simulink model "scars_model_sensors"  (R2019b)
settings: Solver=FixedStepAuto  StartTime=0.0  StopTime=3500  FixedStep=dT  MaxStep=1  MinStep=dT  RelTol=1e-3
model workspace (MAT data in the model file):
  actuators = 0
values from neighbouring files (symbols this model uses):
  dtStep = 10    [SCARSSetup.m]    (also in pwsat2_setup.m; scars_setup.m)
  forcesBody = [0 0 0]    [SCARSSetup.m]    (also in pwsat2_setup.m; scars_setup.m)
  initEuler = [0 0 0]    [SCARSSetup.m]    (also in pwsat2_setup.m; scars_setup.m)
  initMoments = [0 0 0]    [SCARSSetup.m]    (also in pwsat2_setup.m; scars_setup.m)
  momentsBody = [0 0 0]    [SCARSSetup.m]    (also in pwsat2_setup.m; scars_setup.m)
  refEuler = [0 0 1]    [SCARSSetup.m]    (also in pwsat2_setup.m = [0 deg2rad(45) deg2rad(45)]; scars_setup.m)
  refVel = [v_b(1) v_b(2) v_b(3)]    [SCARSSetup.m]    (also in pwsat2_setup.m; scars_setup.m)
  stepTime = 50    [SCARSSetup.m]    (also in pwsat2_setup.m; scars_setup.m)
undefined symbols (not defined in the file or in its folder): bb, Earth, rw, WGS84
libraries: scars_library x7, aerolibgravity2 x2, aerolib6dof2 x1, sharedtransform x1, aerolibutil x1
settings Model: OrderedModelArguments=off  Creator=asmialek  LastModifiedBy=asmialek
settings DataIOCC: SaveFormat=Array  ReturnWorkspaceOutputsName=scars_out

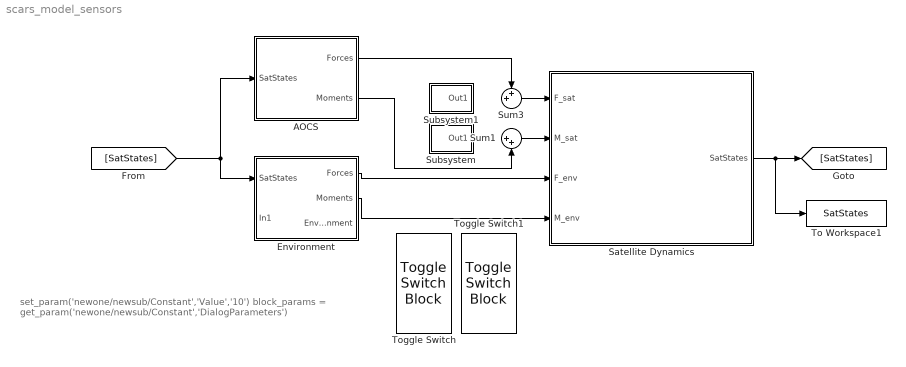
== system scars_model_sensors ==
  note: set_param('newone/newsub/Constant','Value','10')
      |
      |  block_params = get_param('newone/newsub/Constant','DialogParameters')
  AOCS : Subsystem
  Environment : Subsystem
  Satellite Dynamics : Subsystem
  Subsystem : Subsystem
  Subsystem1 : Subsystem
  Sum1 : Sum  Inputs=|++
  Sum3 : Sum  Inputs=++|
  To Workspace1 : ToWorkspace  VariableName=SatStates  SaveFormat=Timeseries  SampleTime=-1
  Toggle Switch : ToggleSwitchBlock
      settings: Values={{'Off', 'On'}, [0 1]}
  Toggle Switch1 : ToggleSwitchBlock
      settings: Values={{'Off', 'On'}, [0 1]}
  wires:
  Satellite Dynamics/1(SatStates) -> To Workspace1/1, [SatStates]
  [SatStates] -> Environment/1(SatStates), AOCS/1(SatStates)
  Environment/1(Forces) -> Satellite Dynamics/3(F_env)
  Environment/2(Moments) -> Satellite Dynamics/4(M_env)
  Sum3/1 -> Satellite Dynamics/1(F_sat)
  Sum1/1 -> Satellite Dynamics/2(M_sat)
  AOCS/1(Forces) -> Sum3/1
  AOCS/2(Moments) -> Sum1/2

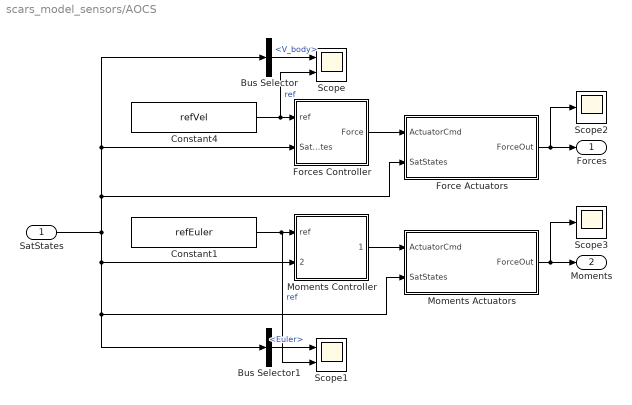
== system scars_model_sensors/AOCS ==
  SatStates : Inport
  Bus Selector : BusSelector  OutputSignals=V_body
  Bus Selector1 : BusSelector  OutputSignals=Euler
  Constant1 : Constant  Value=refEuler
  Constant4 : Constant  Value=refVel
  Force Actuators : Subsystem  mask{ActuatorType=Thrusters}
      mask prompts: ActuatorType "Actuator Type"
      mask TypeOptions ActuatorType: Thrusters | None
      mask Callback ActuatorType:
      | value = get_param(gcb,'ActuatorType');
      | % disp(value);
      | if strcmp(value,'Perfect')
      |     assignin('base','actuators',1)
      | elseif strcmp(value,'Thrusters')
      |     assignin('base','actuators',2)
      | elseif strcmp(value,'None')
      |     assignin('base','actuators',4)
      | else
      |     assignin('base','actuators',4)
      | end
  Forces Controller : Subsystem
  Moments Actuators : Subsystem  mask{ActuatorType=Thrusters}
      mask prompts: ActuatorType "Actuator Type"
      mask TypeOptions ActuatorType: Thrusters | None
      mask Callback ActuatorType:
      | value = get_param(gcb,'ActuatorType');
      | % disp(value);
      | if strcmp(value,'Perfect')
      |     assignin('base','actuators',1)
      | elseif strcmp(value,'Thrusters')
      |     assignin('base','actuators',2)
      | elseif strcmp(value,'None')
      |     assignin('base','actuators',4)
      | else
      |     assignin('base','actuators',4)
      | end
  Moments Controller : Subsystem
  Scope : Scope  NumInputPorts=2
  Scope1 : Scope  NumInputPorts=2
  Scope2 : Scope
  Scope3 : Scope
  Forces : Outport
  Moments : Outport  Port=2
  wires:
  Moments Controller/1(Torque) -> Moments Actuators/1(ActuatorCmd)
  Force Actuators/1(ForceOut) -> Scope2/1, Forces/1
  SatStates/1 -> Bus Selector1/1, Moments Actuators/2(SatStates), Moments Controller/2(SatStates), Bus Selector/1, Forces Controller/2(SatStates), Force Actuators/2(SatStates)
  Constant4/1 -> Scope/2, Forces Controller/1(ref)  "ref"
  Forces Controller/1(Force) -> Force Actuators/1(ActuatorCmd)
  Constant1/1 -> Scope1/2, Moments Controller/1(ref)  "ref"
  Bus Selector/1 -> Scope/1  "<V_body>"
  Bus Selector1/1 -> Scope1/1  "<Euler>"
  Moments Actuators/1(ForceOut) -> Scope3/1, Moments/1

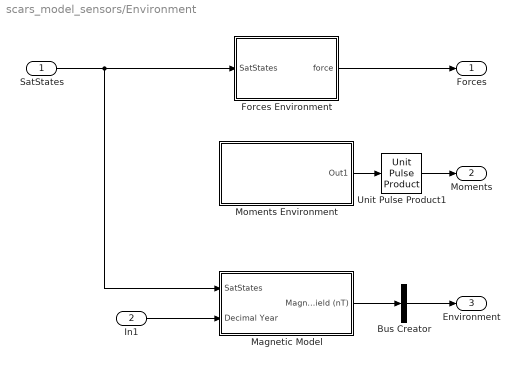
== system scars_model_sensors/Environment ==
  SatStates : Inport
  In1 : Inport  Port=2
  Bus Creator : BusCreator  Inputs=1
  Forces Environment : Subsystem
  Magnetic Model : Subsystem
  Moments Environment : Subsystem
  Unit Pulse Product1 : scars_library/Unit Pulse Product  startTime=stepTime  length=dtStep
  Forces : Outport
  Moments : Outport  Port=2
  Environment : Outport  Port=3
  wires:
  Moments Environment/1(Out1) -> Unit Pulse Product1/1
  SatStates/1 -> Magnetic Model/1(SatStates), Forces Environment/1(SatStates)
  Forces Environment/1(force) -> Forces/1
  Unit Pulse Product1/1 -> Moments/1
  Magnetic Model/1(Magnetic Field (nT)) -> Bus Creator/1
  Bus Creator/1 -> Environment/1
  In1/1 -> Magnetic Model/2(Decimal Year)

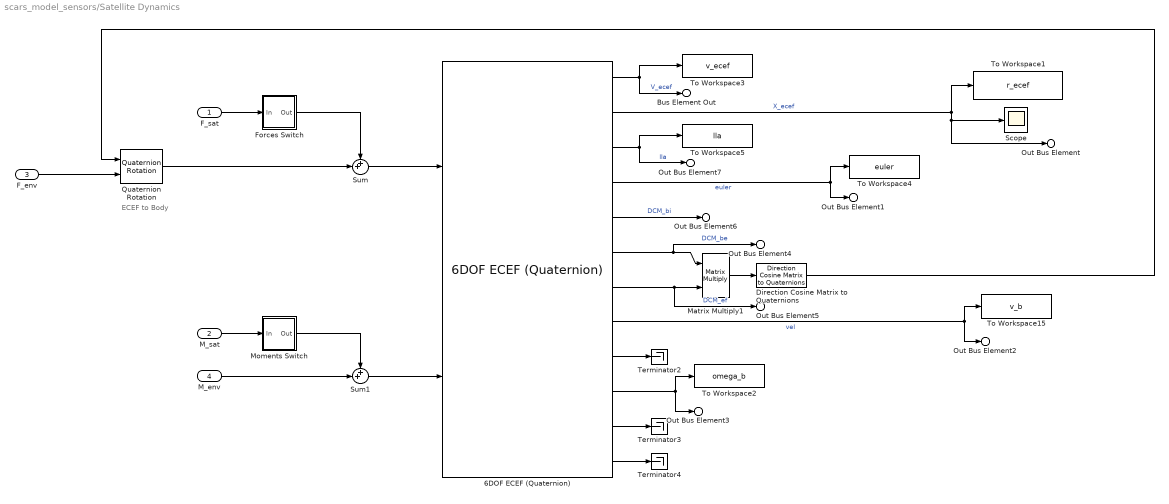
== system scars_model_sensors/Satellite Dynamics ==
  note: ECEF to Body
  F_sat : Inport
  M_sat : Inport  Port=2
  F_env : Inport  Port=3
  M_env : Inport  Port=4
  6DOF ECEF (Quaternion) : aerolib6dof2/6DOF ECEF (Quaternion)  units=Metric (MKS)  mtype=Fixed  xg_0=r_lla  Vm_0=v_b  eul_0=deg2rad(initEuler)  pm_0=[0 0 0]  mass_0=1.0  mass_e=0.5  mass_f=2.0  inertia=eye(3)  inertia_e=eye(3)  inertia_f=2*eye(3)  vre_flag=on  abi_flag=off  ptype=Earth (WGS84)  R=6378137  F=1/298.257223563  w_E=7292115e-11  angle_in=Internal  LG0=0  quat_statename=''  pm_statename=''  Vm_statename=''  posECEF_statename=''  posECI_statename=''  LG_statename=''  mass_statename=''
      settings: SourceProductName=Aerospace Blockset  SourceProductBaseCode=AE
  Direction Cosine Matrix to Quaternions : sharedtransform/Direction Cosine Matrix  to Quaternions  aMode=0  action=None  tolerance=eps(2)
      settings: SourceProductName=Aerospace Blockset  SourceProductBaseCode=AE
  Forces Switch : Subsystem
  Matrix Multiply1 : Product  Multiplication=Matrix(*)
  Moments Switch : Subsystem
  Quaternion Rotation : aerolibutil/Quaternion Rotation
  Scope : Scope
  Sum : Sum  Inputs=++|
  Sum1 : Sum  Inputs=++|
  Terminator2 : Terminator
  Terminator3 : Terminator
  Terminator4 : Terminator
  To Workspace1 : ToWorkspace  VariableName=r_ecef  SampleTime=-1
  To Workspace15 : ToWorkspace  VariableName=v_b  SampleTime=-1
      settings: Save2DSignal=2-D array (concatenate along first dimension)
  To Workspace2 : ToWorkspace  VariableName=omega_b  SampleTime=-1
      settings: Save2DSignal=2-D array (concatenate along first dimension)
  To Workspace3 : ToWorkspace  VariableName=v_ecef  SampleTime=-1
      settings: Save2DSignal=2-D array (concatenate along first dimension)
  To Workspace4 : ToWorkspace  VariableName=euler  SampleTime=-1
      settings: Save2DSignal=2-D array (concatenate along first dimension)
  To Workspace5 : ToWorkspace  VariableName=lla  SampleTime=-1
      settings: Save2DSignal=2-D array (concatenate along first dimension)
  Bus Element Out : Outport  PortName=SatStates  Element=V_ecef
  Out Bus Element : Outport  PortName=SatStates  Element=X_ecef
  Out Bus Element1 : Outport  PortName=SatStates  Element=Euler
  Out Bus Element2 : Outport  PortName=SatStates  Element=V_body
  Out Bus Element3 : Outport  PortName=SatStates  Element=Omega_body
  Out Bus Element6 : Outport  PortName=SatStates  Element=ECI2Body
  Out Bus Element4 : Outport  PortName=SatStates  Element=NED2Body
  Out Bus Element5 : Outport  PortName=SatStates  Element=ECEF2NED
  Out Bus Element7 : Outport  PortName=SatStates  Element=lla
  wires:
  6DOF ECEF (Quaternion)/1 -> To Workspace3/1, Bus Element Out/1  "V_ecef"
  6DOF ECEF (Quaternion)/8 -> Out Bus Element2/1, To Workspace15/1  "vel"
  6DOF ECEF (Quaternion)/2 -> Scope/1, Out Bus Element/1, To Workspace1/1  "X_ecef"
  6DOF ECEF (Quaternion)/6 -> Out Bus Element4/1, Matrix Multiply1/1  "DCM_be"
  Sum/1 -> 6DOF ECEF (Quaternion)/1
  6DOF ECEF (Quaternion)/7 -> Out Bus Element5/1, Matrix Multiply1/2  "DCM_ef"
  6DOF ECEF (Quaternion)/4 -> Out Bus Element1/1, To Workspace4/1  "euler"
  6DOF ECEF (Quaternion)/10 -> To Workspace2/1, Out Bus Element3/1
  M_env/1 -> Sum1/2
  Sum1/1 -> 6DOF ECEF (Quaternion)/2
  Matrix Multiply1/1 -> Direction Cosine Matrix to Quaternions/1
  F_sat/1 -> Forces Switch/1(In)
  Quaternion Rotation/1 -> Sum/2
  F_env/1 -> Quaternion Rotation/2
  Direction Cosine Matrix to Quaternions/1 -> Quaternion Rotation/1
  Forces Switch/1(Out) -> Sum/1
  M_sat/1 -> Moments Switch/1(In)
  Moments Switch/1(Out) -> Sum1/1
  6DOF ECEF (Quaternion)/5 -> Out Bus Element6/1  "DCM_bi"
  6DOF ECEF (Quaternion)/9 -> Terminator2/1
  6DOF ECEF (Quaternion)/11 -> Terminator3/1
  6DOF ECEF (Quaternion)/12 -> Terminator4/1
  6DOF ECEF (Quaternion)/3 -> Out Bus Element7/1, To Workspace5/1  "lla"

== system scars_model_sensors/Subsystem ==
  Constant1 : Constant  Value=momentsBody
  Constant2 : Constant  Value=momentsBody
  Gain : Gain  Gain=-1
  Sum : Sum  Inputs=|++
  Unit Pulse Product1 : scars_library/Unit Pulse Product  startTime=stepTime  length=dtStep
  Unit Pulse Product2 : scars_library/Unit Pulse Product  startTime=stepTime+dtStep  length=dtStep
  Out1 : Outport
  wires:
  Constant1/1 -> Unit Pulse Product1/1
  Unit Pulse Product1/1 -> Sum/1
  Sum/1 -> Out1/1
  Constant2/1 -> Unit Pulse Product2/1
  Gain/1 -> Sum/2
  Unit Pulse Product2/1 -> Gain/1

== system scars_model_sensors/Subsystem1 ==
  Constant2 : Constant  Value=forcesBody
  Unit Pulse Product : scars_library/Unit Pulse Product  startTime=stepTime+100  length=dtStep
  Out1 : Outport
  wires:
  Constant2/1 -> Unit Pulse Product/1
  Unit Pulse Product/1 -> Out1/1

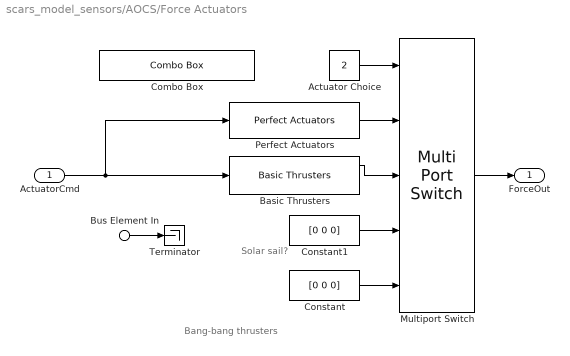
== system scars_model_sensors/AOCS/Force Actuators ==
  note: Bang-bang thrusters
  note: Solar sail?
  ActuatorCmd : Inport
  Bus Element In : Inport  Port=2  PortName=SatStates  Element=V_ecef
  Actuator Choice : Constant  Value=2
  Basic Thrusters : scars_library/Basic Thrusters  SystemSampleTime=-1  Latency=0  AutoFrameSizeCalculation=off
  Combo Box : ComboBox  LabelPosition=Hide  SelectedLabel=Thrusters
      settings: Values={{'Perfect Actuators', 'Thrusters', 'idontknowyet', 'No Actuators'}, [1 2 3 4]}
  Constant : Constant  Value=[0 0 0]
  Constant1 : Constant  Value=[0 0 0]
  Multiport Switch : MultiPortSwitch  Inputs=4  DiagnosticForDefault=Warning
  Perfect Actuators : scars_library/Perfect Actuators  Parameter1=on
  Terminator : Terminator
  ForceOut : Outport
  wires:
  Perfect Actuators/1 -> Multiport Switch/2
  Constant/1 -> Multiport Switch/5
  Actuator Choice/1 -> Multiport Switch/1
  Basic Thrusters/1 -> Multiport Switch/3
  ActuatorCmd/1 -> Basic Thrusters/1, Perfect Actuators/1
  Multiport Switch/1 -> ForceOut/1
  Constant1/1 -> Multiport Switch/4
  Bus Element In/1 -> Terminator/1

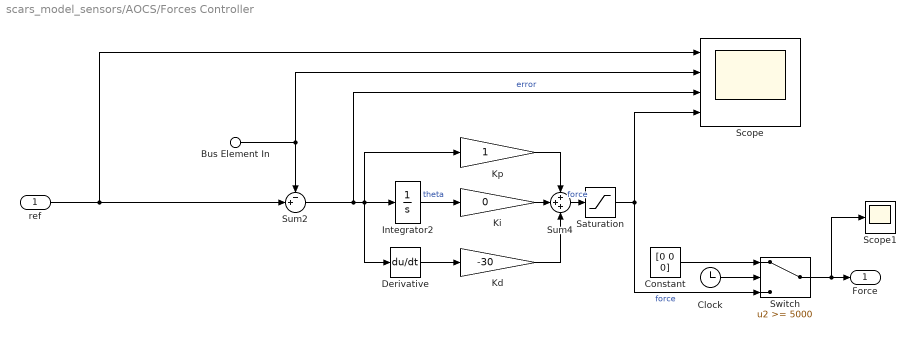
== system scars_model_sensors/AOCS/Forces Controller ==
  ref : Inport
  Bus Element In : Inport  Port=2  PortName=SatStates  Element=V_body
  Clock : Clock
  Constant : Constant  Value=[0 0 0]
  Derivative : Derivative
  Integrator2 : Integrator
  Kd : Gain  Gain=-30
  Ki : Gain  Gain=0
  Kp : Gain
  Saturation : Saturate
  Scope : Scope  NumInputPorts=4
  Scope1 : Scope
  Sum2 : Sum  Inputs=-+|
  Sum4 : Sum  Inputs=+++
  Switch : Switch  Threshold=5000
  Force : Outport
  wires:
  Saturation/1 -> Switch/3, Scope/4  "force"
  ref/1 -> Sum2/2, Scope/1
  Clock/1 -> Switch/2
  Switch/1 -> Scope1/1, Force/1
  Constant/1 -> Switch/1
  Bus Element In/1 -> Sum2/1, Scope/2
  Integrator2/1 -> Ki/1  "theta"
  Kp/1 -> Sum4/1
  Sum2/1 -> Kp/1, Derivative/1, Integrator2/1, Scope/3  "error"
  Kd/1 -> Sum4/3
  Ki/1 -> Sum4/2
  Derivative/1 -> Kd/1
  Sum4/1 -> Saturation/1  "force"

== system scars_model_sensors/AOCS/Moments Actuators ==
  ActuatorCmd : Inport
  Bus Element In : Inport  Port=2  PortName=SatStates  Element=Euler
  Actuator Choice : Constant  Value=2
  Bang-Bang Thrusters : Subsystem
  Constant : Constant  Value=[0 0 0]
  Multiport Switch : MultiPortSwitch  Inputs=4  DiagnosticForDefault=Warning
  Perfect Actuators : scars_library/Perfect Actuators  Parameter1=on
  Reaction Wheels : Subsystem
  ForceOut : Outport
  wires:
  Perfect Actuators/1 -> Multiport Switch/2
  Constant/1 -> Multiport Switch/5
  Actuator Choice/1 -> Multiport Switch/1
  Bang-Bang Thrusters/1(Torque) -> Multiport Switch/3
  Reaction Wheels/1(Torque) -> Multiport Switch/4
  Multiport Switch/1 -> ForceOut/1
  ActuatorCmd/1 -> Bang-Bang Thrusters/1(TorqueCmd), Perfect Actuators/1, Reaction Wheels/2(TorqueCmd)
  Bus Element In/1 -> Reaction Wheels/1(Euler)

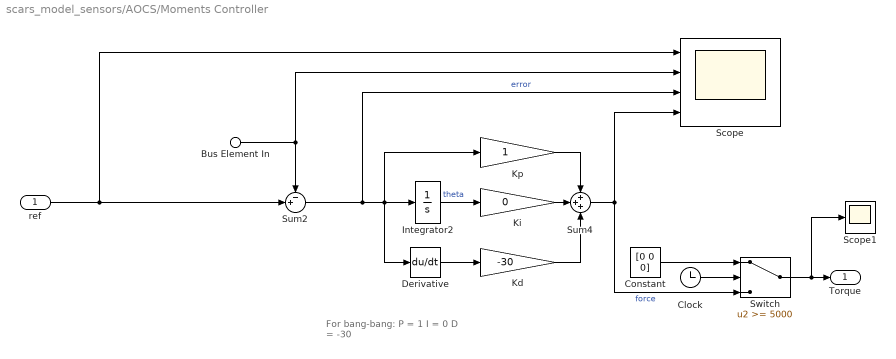
== system scars_model_sensors/AOCS/Moments Controller ==
  note: For bang-bang:
      | P = 1
      | I = 0
      | D = -30
  ref : Inport
  Bus Element In : Inport  Port=2  PortName=SatStates  Element=Euler
  Clock : Clock
  Constant : Constant  Value=[0 0 0]
  Derivative : Derivative
  Integrator2 : Integrator
  Kd : Gain  Gain=-30
  Ki : Gain  Gain=0
  Kp : Gain
  Scope : Scope  NumInputPorts=4
  Scope1 : Scope
  Sum2 : Sum  Inputs=-+|
  Sum4 : Sum  Inputs=+++
  Switch : Switch  Threshold=5000
  Torque : Outport
  wires:
  Sum4/1 -> Switch/3, Scope/4  "force"
  ref/1 -> Sum2/2, Scope/1
  Clock/1 -> Switch/2
  Switch/1 -> Scope1/1, Torque/1
  Constant/1 -> Switch/1
  Bus Element In/1 -> Sum2/1, Scope/2
  Derivative/1 -> Kd/1
  Kd/1 -> Sum4/3
  Ki/1 -> Sum4/2
  Integrator2/1 -> Ki/1  "theta"
  Sum2/1 -> Kp/1, Derivative/1, Integrator2/1, Scope/3  "error"
  Kp/1 -> Sum4/1

== system scars_model_sensors/Environment/Forces Environment ==
  Bus Element In : Inport  PortName=SatStates  Element=X_ecef
  Spherical Harmonic Gravity Model1 : aerolibgravity2/Spherical Harmonic Gravity Model  units=Metric (MKS)  degree=120  action=Warning  ptype=EGM2008  datafile='aerogmm2b.mat'
      settings: SourceProductName=Aerospace Blockset  SourceProductBaseCode=AE
  To Workspace13 : ToWorkspace  VariableName=g  SampleTime=-1
  force : Outport
  wires:
  Spherical Harmonic Gravity Model1/1 -> force/1, To Workspace13/1
  Bus Element In/1 -> Spherical Harmonic Gravity Model1/1

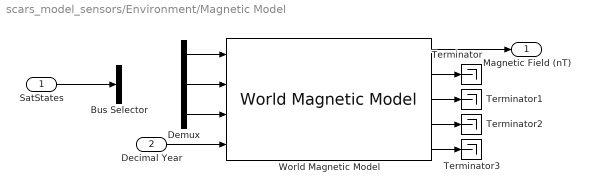
== system scars_model_sensors/Environment/Magnetic Model ==
  SatStates : Inport
  Decimal Year : Inport  Port=2
  Bus Selector : BusSelector  OutputSignals=signal1,signal2
  Demux : Demux  Outputs=3
  Terminator{,1..3} (4 alike) : Terminator
  World Magnetic Model : aerolibgravity2/World Magnetic Model  model=WMM2015 V2 (2015-2020)  customFile='WMM2015v2.COF'  units=Metric (MKS)  time_in=on  month=January  day=1  year=2015  action=Error  h_out=on  dec_out=on  inc_out=on  ti_out=on
      settings: SourceProductName=Aerospace Blockset  SourceProductBaseCode=AE
  Magnetic Field (nT) : Outport
  wires:
  World Magnetic Model/4 -> Terminator2/1
  Demux/1 -> World Magnetic Model/1
  World Magnetic Model/1 -> Magnetic Field (nT)/1
  Demux/3 -> World Magnetic Model/3
  Decimal Year/1 -> World Magnetic Model/4
  World Magnetic Model/2 -> Terminator/1
  World Magnetic Model/5 -> Terminator3/1
  World Magnetic Model/3 -> Terminator1/1
  Demux/2 -> World Magnetic Model/2
  SatStates/1 -> Bus Selector/1

== system scars_model_sensors/Environment/Moments Environment ==
  Constant : Constant  Value=initMoments
  Out1 : Outport
  wires:
  Constant/1 -> Out1/1

== system scars_model_sensors/Satellite Dynamics/Forces Switch ==
  In : Inport
  Constant1 : Constant  Value=[0 0 0]
  Forces : Constant  Value=0
  Switch : Switch  Criteria=u2 > Threshold
  Out : Outport
  wires:
  Constant1/1 -> Switch/3
  Forces/1 -> Switch/2
  Switch/1 -> Out/1
  In/1 -> Switch/1

== system scars_model_sensors/Satellite Dynamics/Moments Switch ==
  In : Inport
  Constant1 : Constant  Value=[0 0 0]
  Moments : Constant  Value=0
  Switch : Switch  Criteria=u2 > Threshold
  Out : Outport
  wires:
  In/1 -> Switch/1
  Constant1/1 -> Switch/3
  Switch/1 -> Out/1
  Moments/1 -> Switch/2

== system scars_model_sensors/AOCS/Moments Actuators/Bang-Bang Thrusters ==
  TorqueCmd : Inport
  Demux : Demux  Outputs=3
  Gain : Gain  Gain=-1
  Mux : Mux  Inputs=3
  Thruster Pitch : Subsystem
  Thruster Roll : Subsystem
  Thruster Yaw : Subsystem
  Torque : Outport  VectorParamsAs1DForOutWhenUnconnected=off
  wires:
  Thruster Roll/1(Torque Out) -> Mux/1
  Thruster Pitch/1(Torque Out) -> Mux/2
  Thruster Yaw/1(Torque Out) -> Mux/3
  TorqueCmd/1 -> Demux/1
  Demux/2 -> Thruster Pitch/1(Torque)
  Demux/1 -> Thruster Roll/1(Torque)
  Demux/3 -> Thruster Yaw/1(Torque)
  Mux/1 -> Gain/1
  Gain/1 -> Torque/1

== system scars_model_sensors/AOCS/Moments Actuators/Reaction Wheels ==
  Euler : Inport
  TorqueCmd : Inport  Port=2
  Demux : Demux  Outputs=3
  Demux2 : Demux  Outputs=3
  Mux : Mux  Inputs=3
  Reaction Wheel Pitch : Subsystem
  Reaction Wheel Roll : Subsystem
  Reaction Wheel Yaw : Subsystem
  Torque : Outport  VectorParamsAs1DForOutWhenUnconnected=off
  wires:
  Mux/1 -> Torque/1
  Demux/1 -> Reaction Wheel Roll/2(Torque)
  Reaction Wheel Roll/1(Torque Out) -> Mux/1
  Demux2/1 -> Reaction Wheel Roll/1(Rate)
  Demux2/2 -> Reaction Wheel Pitch/1(Rate)
  Demux/2 -> Reaction Wheel Pitch/2(Torque)
  Demux2/3 -> Reaction Wheel Yaw/1(Rate)
  Demux/3 -> Reaction Wheel Yaw/2(Torque)
  Reaction Wheel Pitch/1(Torque Out) -> Mux/2
  Reaction Wheel Yaw/1(Torque Out) -> Mux/3
  Euler/1 -> Demux2/1
  TorqueCmd/1 -> Demux/1

== system scars_model_sensors/AOCS/Moments Actuators/Bang-Bang Thrusters/Thruster Pitch ==
  Torque : Inport
  Gain2 : Gain  Gain=-1
  Relay1 : Relay  OnSwitchValue=bb.a1  OffSwitchValue=bb.a0  OnOutputValue=bb.thrust
  Relay2 : Relay  OnSwitchValue=bb.a1  OffSwitchValue=bb.a0  OnOutputValue=-bb.thrust
  Scope1 : Scope  NumInputPorts=5
  Sum1 : Sum  Inputs=-|-
  Sum2 : Sum  Inputs=+|+
  Torque Out : Outport
  wires:
  Sum1/1 -> Torque Out/1  "M"
  Relay2/1 -> Scope1/3, Sum2/2
  Sum2/1 -> Scope1/5, Sum1/1
  Gain2/1 -> Scope1/2, Relay2/1
  Relay1/1 -> Scope1/4, Sum2/1
  Torque/1 -> Scope1/1, Relay1/1, Gain2/1  "pd"

== system scars_model_sensors/AOCS/Moments Actuators/Bang-Bang Thrusters/Thruster Roll ==
  Torque : Inport
  Gain2 : Gain  Gain=-1
  Relay1 : Relay  OnSwitchValue=bb.a1  OffSwitchValue=bb.a0  OnOutputValue=bb.thrust
  Relay2 : Relay  OnSwitchValue=bb.a1  OffSwitchValue=bb.a0  OnOutputValue=-bb.thrust
  Scope1 : Scope  NumInputPorts=5
  Sum1 : Sum  Inputs=-|-
  Sum2 : Sum  Inputs=+|+
  Torque Out : Outport
  wires:
  Sum1/1 -> Torque Out/1  "M"
  Relay2/1 -> Scope1/3, Sum2/2
  Sum2/1 -> Scope1/5, Sum1/1
  Gain2/1 -> Scope1/2, Relay2/1
  Relay1/1 -> Scope1/4, Sum2/1
  Torque/1 -> Scope1/1, Relay1/1, Gain2/1  "pd"

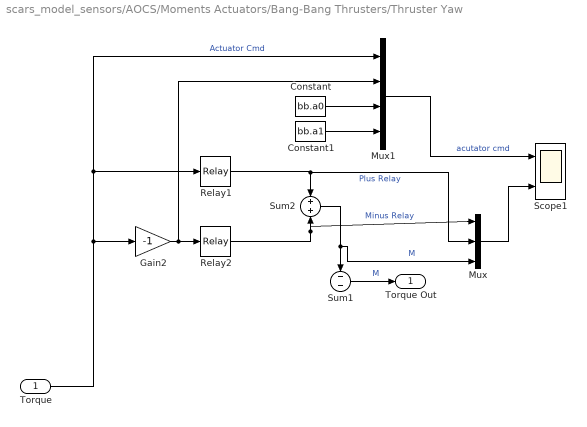
== system scars_model_sensors/AOCS/Moments Actuators/Bang-Bang Thrusters/Thruster Yaw ==
  Torque : Inport
  Constant : Constant  Value=bb.a0
  Constant1 : Constant  Value=bb.a1
  Gain2 : Gain  Gain=-1
  Mux : Mux  Inputs=3
  Mux1 : Mux
  Relay1 : Relay  OnSwitchValue=bb.a1  OffSwitchValue=bb.a0  OnOutputValue=bb.thrust
  Relay2 : Relay  OnSwitchValue=bb.a1  OffSwitchValue=bb.a0  OnOutputValue=-bb.thrust
  Scope1 : Scope  NumInputPorts=2
  Sum1 : Sum  Inputs=-|-
  Sum2 : Sum  Inputs=+|+
  Torque Out : Outport
  wires:
  Sum1/1 -> Torque Out/1  "M"
  Relay2/1 -> Mux/1, Sum2/2  "Minus Relay"
  Sum2/1 -> Mux/3, Sum1/1  "M"
  Gain2/1 -> Mux1/2, Relay2/1
  Relay1/1 -> Mux/2, Sum2/1  "Plus Relay"
  Torque/1 -> Relay1/1, Mux1/1, Gain2/1  "Actuator Cmd"
  Mux1/1 -> Scope1/1  "acutator cmd"
  Mux/1 -> Scope1/2
  Constant/1 -> Mux1/3
  Constant1/1 -> Mux1/4

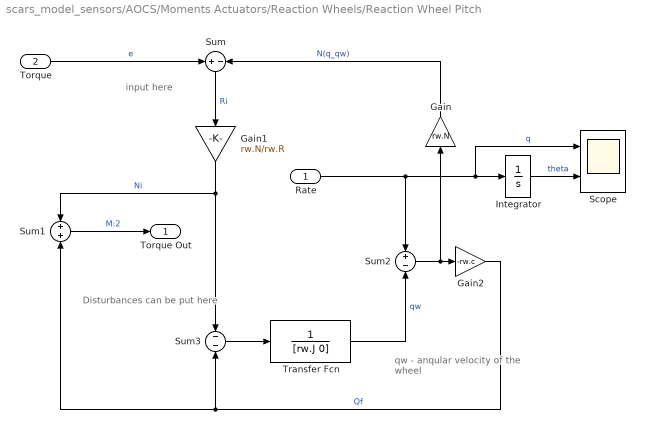
== system scars_model_sensors/AOCS/Moments Actuators/Reaction Wheels/Reaction Wheel Pitch ==
  note: qw - anqular velocity
      |  of the wheel
  note: input here
  note: Disturbances can
      | be put here
  Rate : Inport
  Torque : Inport  Port=2
  Gain : Gain  Gain=rw.N
  Gain1 : Gain  Gain=rw.N/rw.R
  Gain2 : Gain  Gain=-rw.c
  Integrator : Integrator
  Scope : Scope  NumInputPorts=2
  Sum : Sum  Inputs=+|-
  Sum1 : Sum  Inputs=+|+
  Sum2 : Sum  Inputs=+|-
  Sum3 : Sum  Inputs=-|-
  Transfer Fcn : TransferFcn  Denominator=[rw.J 0]
  Torque Out : Outport
  wires:
  Gain2/1 -> Sum1/2, Sum3/2  "Qf"
  Gain1/1 -> Sum1/1, Sum3/1  "Ni"
  Integrator/1 -> Scope/2  "theta"
  Sum3/1 -> Transfer Fcn/1
  Torque/1 -> Sum/1  "e"
  Sum1/1 -> Torque Out/1  "M:2"
  Gain/1 -> Sum/2  "N(q_qw)"
  Rate/1 -> Sum2/1, Integrator/1, Scope/1  "q"
  Sum2/1 -> Gain/1, Gain2/1
  Sum/1 -> Gain1/1  "Ri"
  Transfer Fcn/1 -> Sum2/2  "qw"

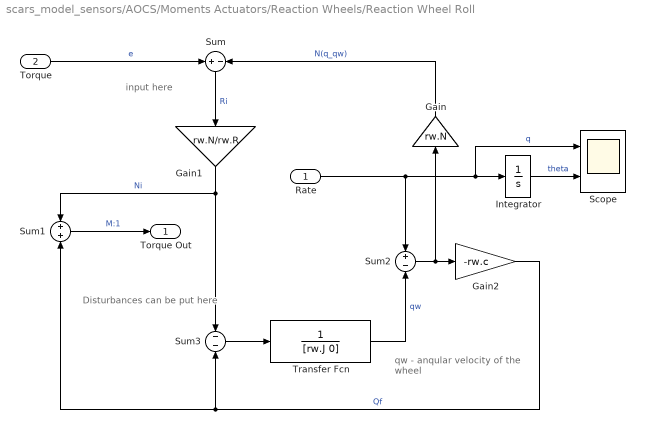
== system scars_model_sensors/AOCS/Moments Actuators/Reaction Wheels/Reaction Wheel Roll ==
  note: Disturbances can
      | be put here
  note: input here
  note: qw - anqular velocity
      |  of the wheel
  Rate : Inport
  Torque : Inport  Port=2
  Gain : Gain  Gain=rw.N
  Gain1 : Gain  Gain=rw.N/rw.R
  Gain2 : Gain  Gain=-rw.c
  Integrator : Integrator
  Scope : Scope  NumInputPorts=2
  Sum : Sum  Inputs=+|-
  Sum1 : Sum  Inputs=+|+
  Sum2 : Sum  Inputs=+|-
  Sum3 : Sum  Inputs=-|-
  Transfer Fcn : TransferFcn  Denominator=[rw.J 0]
  Torque Out : Outport
  wires:
  Gain1/1 -> Sum1/1, Sum3/1  "Ni"
  Torque/1 -> Sum/1  "e"
  Sum3/1 -> Transfer Fcn/1
  Sum/1 -> Gain1/1  "Ri"
  Integrator/1 -> Scope/2  "theta"
  Transfer Fcn/1 -> Sum2/2  "qw"
  Gain2/1 -> Sum1/2, Sum3/2  "Qf"
  Sum1/1 -> Torque Out/1  "M:1"
  Sum2/1 -> Gain2/1, Gain/1
  Gain/1 -> Sum/2  "N(q_qw)"
  Rate/1 -> Sum2/1, Integrator/1, Scope/1  "q"

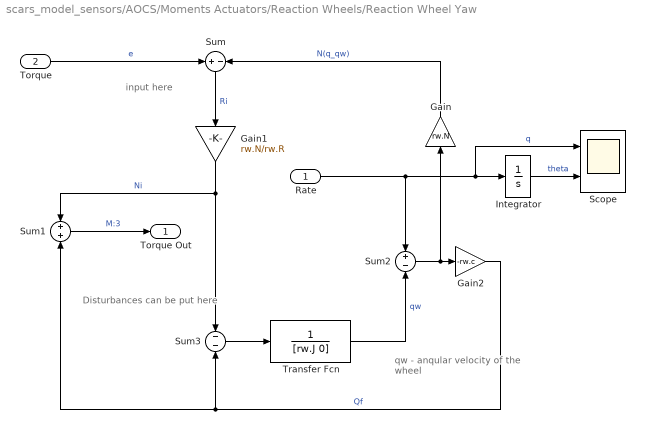
== system scars_model_sensors/AOCS/Moments Actuators/Reaction Wheels/Reaction Wheel Yaw ==
  note: qw - anqular velocity
      |  of the wheel
  note: input here
  note: Disturbances can
      | be put here
  Rate : Inport
  Torque : Inport  Port=2
  Gain : Gain  Gain=rw.N
  Gain1 : Gain  Gain=rw.N/rw.R
  Gain2 : Gain  Gain=-rw.c
  Integrator : Integrator
  Scope : Scope  NumInputPorts=2
  Sum : Sum  Inputs=+|-
  Sum1 : Sum  Inputs=+|+
  Sum2 : Sum  Inputs=+|-
  Sum3 : Sum  Inputs=-|-
  Transfer Fcn : TransferFcn  Denominator=[rw.J 0]
  Torque Out : Outport
  wires:
  Gain2/1 -> Sum1/2, Sum3/2  "Qf"
  Gain1/1 -> Sum1/1, Sum3/1  "Ni"
  Integrator/1 -> Scope/2  "theta"
  Sum3/1 -> Transfer Fcn/1
  Torque/1 -> Sum/1  "e"
  Sum1/1 -> Torque Out/1  "M:3"
  Gain/1 -> Sum/2  "N(q_qw)"
  Rate/1 -> Sum2/1, Integrator/1, Scope/1  "q"
  Sum2/1 -> Gain/1, Gain2/1
  Sum/1 -> Gain1/1  "Ri"
  Transfer Fcn/1 -> Sum2/2  "qw"
